simulink model "ATOM_planning_sim_variable_rear_ratio"  (R2026a)
settings: Solver=ode4  FixedStep=0.01
model workspace (MAT data in the model file):
  vehicle : object (value not decoded)
symbols that are objects in the model workspace (value not decoded): vehicle
undefined symbols (not defined in the file or in its folder): planning_validator, stanley, velocity_smoother
(part 2 of 4)

== matlab function ATOM_planning_sim_variable_rear_ratio/velocity_smoother_node/ApplySteeringRateLimit - velocity_smoother_node/Step2: Calculate steer rate for each trajectory point/ComputeSteeringRate4WS ==
  data: trajectory input Bus: TrajectoryDataBus; curvature input; veh input; steer_rate_velocity_ratio_arr output; points_interval input; output output Bus: TrajectoryDataBus
function [steer_rate_velocity_ratio_arr, output] = ComputeSteeringRateAngle4WS(trajectory, ...
    curvature, veh, ...
    points_interval)


% ComputeSteeringRateAngle4WS
%
% Computes steering angle rate ratio for 4WS.
%
% Equivalent to Autoware:
%
% steer_rate_velocity_ratio_arr
%
%
% The returned value represents:
%
%       steering_angle_difference / distance
%
%
% For 4WS:
%
% front and rear steering rates are computed.
%
% The maximum steering variation is used as constraint.

wheel_base = veh(3);
rear_steering_ratio = veh(29);

N = length(curvature);


front_angle = zeros(N,1);
rear_angle  = zeros(N,1);


%% Compute steering angles

for i = 1:N

    front_angle(i)= ...                                         % Modified for 4WS
        CalculateFrontSteeringAngle4WS( ...
        curvature(i), ...
        wheel_base, ...
        rear_steering_ratio);

    rear_angle(i) = rear_steering_ratio * front_angle(i);       % Modified for 4WS


    % This is a collateral effect of (&) in C++ when (considering in original
    % Autoware):
    %
    % auto & steer_front = output.at(i + 1).front_wheel_angle_rad;
    % auto & steer_back = output.at(i).front_wheel_angle_rad;
    % 
    % // calculate the just 2 steering angle
    % steer_front = std::atan(base_param_.wheel_base * curvature_v.at(i + 1));
    % steer_back = std::atan(base_param_.wheel_base * curvature_v.at(i));
    % Indeed, updating steer_front we popolate also output.at(i + 1).front_wheel_angle_rad, 
    % and so the output topic is populated (but it's just a collateral effect, front_wheel_angle_rad 
    % and rear_wheel_angle_rad contents are not important for Control module.

    trajectory.front_wheel_angle_rad(i) = front_angle(i);
    trajectory.rear_wheel_angle_rad(i) = rear_angle(i);

end




%% Compute steering rate

steer_rate_velocity_ratio_arr = zeros(N,1);


for i = 1:N-1


    % auto & steer_front = output.at(i + 1).front_wheel_angle_rad;
    % auto & steer_back = output.at(i).front_wheel_angle_rad;
    % const auto steering_diff = std::fabs(steer_front - steer_back);
    front_diff = abs( ...
        front_angle(i+1)-front_angle(i));


    rear_diff = abs( ...
        rear_angle(i+1)-rear_angle(i));


    steering_diff = max( ...                                    % Modified for 4WS --> conservative solution
        front_diff,...
        rear_diff);

    % eps avoids division by zero:
    eps = 2.220446049250313e-16;

    steer_rate_velocity_ratio_arr(i)= ...
        steering_diff/(points_interval+eps);


end


steer_rate_velocity_ratio_arr(end)= ...
    steer_rate_velocity_ratio_arr(end-1);


% Output topic now presents front_wheel_angle_rad and rear_wheel_angle_rad
% populated
output = trajectory;


end

== matlab function ATOM_planning_sim_variable_rear_ratio/velocity_smoother_node/ApplySteeringRateLimit - velocity_smoother_node/Step3: Remove noise by mean filter/MeanFilterSteeringRateRato ==
  data: steer_rate_ratio input; steer_rate_velocity_ratio_arr output
function steer_rate_velocity_ratio_arr = MeanFilterSteeringRateRatio( ...
    steer_rate_ratio)

% MeanFilterSteeringRateRatio
%
% Applies the same moving-average filter used by Autoware on the steering
% rate ratio.
%
% Equivalent to Step 3 inside:
%
%   SmootherBase::applySteeringRateLimit()
%
% in:
%
%   autoware_velocity_smoother
%
%
% Original C++ implementation:
%
% for (size_t i = 1; i < steer_rate_velocity_ratio_arr.size() - 1; i++) {
%
%   steer_rate_velocity_ratio_arr.at(i) =
%     (steer_rate_velocity_ratio_arr.at(i-1) +
%      steer_rate_velocity_ratio_arr.at(i)   +
%      steer_rate_velocity_ratio_arr.at(i+1))
%      / 3.0;
%
% }
%
%
% Notes
% -----
%
% The filter is performed in-place, exactly as in Autoware.
%
% Consequently, when computing sample i, the previous sample
% (i-1) has already been filtered, while the next sample (i+1)
% is still the original one.
%
% This behaviour is intentionally preserved to remain identical
% to the C++ implementation.


N = length(steer_rate_ratio);

steer_rate_velocity_ratio_arr = zeros(N,1);

for i = 2:N-1

    steer_rate_velocity_ratio_arr(i) = ...
        ( ...
        steer_rate_ratio(i-1) + ...
        steer_rate_ratio(i)   + ...
        steer_rate_ratio(i+1) ...
        ) / 3.0;

end


end

== matlab function ATOM_planning_sim_variable_rear_ratio/velocity_smoother_node/ApplySteeringRateLimit - velocity_smoother_node/ComputePointsInterval ==
  data: input_points_interval input; vel_smoother input; use_resampling input; points_interval output
function points_interval = computePointsInterval(input_points_interval, ...
    vel_smoother, use_resampling)

% Compute the trajectory points interval used for preprocessing.
%
% If resampling is enabled, a constant spatial interval is imposed.
% Otherwise, the original trajectory point spacing is preserved.

sample_ds = vel_smoother(3,1);

if use_resampling

    points_interval = sample_ds;

else

    points_interval = input_points_interval;

end

end

== matlab function ATOM_planning_sim_variable_rear_ratio/velocity_smoother_node/ApplySteeringRateLimit - velocity_smoother_node/ComputeIdxDist ==
  data: points_interval input; idx_dist output; vel_smoother input
function idx_dist = ComputeIdxDist( ...
    points_interval, ...
    vel_smoother)

% ComputeIdxDist
%
% Computes the point offset used for trajectory curvature estimation.
%
% The curvature is evaluated using three trajectory points separated by a
% fixed physical distance. Since the trajectory is sampled with a constant
% spatial interval (points_interval), this function converts the desired
% curvature calculation distance into the corresponding point index offset.
%
% In other words, idx_dist represents the number of trajectory points
% corresponding to the specified curvature calculation distance.
%
% Equivalent to the Autoware implementation:
%
% idx_dist = max(int(curvature_calculation_distance / points_interval), 1);

curvature_calculation_distance = vel_smoother(1);

idx_dist = max( ...
    floor(curvature_calculation_distance / points_interval), ...
    1);

== matlab function ATOM_planning_sim_variable_rear_ratio/velocity_smoother_node/ApplySteeringRateLimit - velocity_smoother_node/PlotTrajectoryCurvature ==
  data: trajectory input; curvature input
function PlotTrajectoryCurvature(trajectory, curvature)

% PlotTrajectoryCurvature
%
% Visualizes the trajectory curvature computed by:
%
%   ComputeTrajectoryCurvature()
%
% Equivalent to inspecting:
%
%   std::vector<double> k_arr
%
% generated inside:
%
%   autoware_motion_utils::calcTrajectoryCurvatureFrom3Points()
%
%
% Inputs
% -------
%
% trajectory:
%   MATLAB representation of Autoware TrajectoryPoints:
%
%       trajectory.pose.position.x
%       trajectory.pose.position.y
%
%
% curvature:
%   Nx1 signed curvature vector [1/m].
%
%   Positive curvature  -> left turn
%   Negative curvature  -> right turn


persistent hCurvature
persistent hTraj


%% Extract trajectory position

x = trajectory.pose.position.x;
y = trajectory.pose.position.y;


%% Check dimensions

if length(curvature) ~= length(x)

    error("Curvature vector length does not match trajectory length.");

end


%% Curvature profile

if isempty(hCurvature) 

    figure(3)
    clf

    hold on
    grid on

    hCurvature = plot( ...
        curvature, ...
        'LineWidth',1.5);


    xlabel("Trajectory point index");
    ylabel("Curvature [1/m]");

    title("Curvature profile");


else

    set(hCurvature,...
        'YData',curvature);

end



%% XY trajectory colored by curvature

if isempty(hTraj) 

    figure(4)
    clf

    hold on
    grid on
    axis equal


    hTraj = scatter( ...
        x, ...
        y, ...
        25, ...
        curvature, ...
        'filled');


    xlabel("x [m]");
    ylabel("y [m]");

    title("Trajectory curvature map");


    cb = colorbar;
    ylabel(cb,'Curvature [1/m]');


else

    set(hTraj,...
        'XData',x,...
        'YData',y,...
        'CData',curvature);

end


drawnow limitrate


end

== matlab function ATOM_planning_sim_variable_rear_ratio/velocity_smoother_node/ApplySteeringRateLimit - velocity_smoother_node/ComputeSteerRateVelocityRatioLimits ==
  data: velocity_thresholds input; steer_rate_velocity_ratio_limits output; steering_angle_rate_limits input
function steer_rate_velocity_ratio_limits = ...
    ComputeSteerRateVelocityRatioLimits( ...
    velocity_thresholds, ...
    steering_angle_rate_limits)

% ComputeSteerRateVelocityRatioLimits
%
% MATLAB equivalent of:
%
%   SmootherBase::computeSteerRateVelocityRatioLimits()
%
% in Autoware.
%
% It computes the steering-rate / velocity ratio limits used later by
% ComputeVelocityLimitFromSteerRate().
%
%
% Equivalent C++:
%
% return computeRatioLimits<double>(
%     velocity_thresholds,
%     steering_angle_rate_limits,
%     compute_steer_rate_ratio);
%
%
% Inputs
% -------
%
% velocity_thresholds
%       Velocity breakpoints [m/s]
%
% steering_angle_rate_limits
%       Maximum steering rate [deg/s]
%
%
% Output
% ------
%
% steer_rate_velocity_ratio_limits
%
% Nx2 matrix equivalent to:
%
% std::vector<std::pair<double,double>>
%
% Each row contains:
%
%   [ratio_lower , ratio_upper]
%
% corresponding to one velocity interval.


epsilon = 1e-5;

N = length(velocity_thresholds);

steer_rate_velocity_ratio_limits = zeros(N+1,2);


%% Compute ratio limits

for i = 1:N

    rate_deg = steering_angle_rate_limits(i);

    vi = velocity_thresholds(i);

    if i == 1
        vi_prev = 0.0;
    else
        vi_prev = velocity_thresholds(i-1);
    end

    steer_rate_velocity_ratio_limits(i,1) = ...
        deg2rad(rate_deg)/(vi_prev + epsilon);

    steer_rate_velocity_ratio_limits(i,2) = ...
        deg2rad(rate_deg)/(vi + epsilon);

end


%% Last interval

v_max = velocity_thresholds(end);

steer_rate_velocity_ratio_limits(end,1) = ...
    deg2rad(steering_angle_rate_limits(end)) / ...
    (v_max + epsilon);

steer_rate_velocity_ratio_limits(end,2) = 0.0;

end

== matlab function ATOM_planning_sim_variable_rear_ratio/velocity_smoother_node/MATLAB Function ==
  data: trajectory_input input; trajectory_output input; curvature input
function PlotSteeringRateVelocityLimit( ...
    trajectory_input, ...
    trajectory_output, ...
    curvature)

% PlotSteeringRateVelocityLimit
%
% Visualizes the velocity modification produced by the steering-rate
% velocity constraint.
%
% Equivalent to inspecting the difference between:
%
%   input.longitudinal_velocity_mps
%
% and:
%
%   output.longitudinal_velocity_mps
%
% after:
%
%   SmootherBase::applySteeringRateLimit()
%
% in Autoware.
%
%
% The steering-rate filter does not modify the trajectory geometry.
% It only reduces longitudinal velocity where the steering rate
% constraint is violated.
%
%
% Inputs
% -------
%
% trajectory_input:
%       Trajectory before ApplySteeringRateVelocityLimit()
%
%       Required fields:
%           trajectory.longitudinal_velocity_mps
%
%
% trajectory_output:
%       Trajectory after ApplySteeringRateVelocityLimit()
%
%       Required fields:
%           trajectory.longitudinal_velocity_mps
%
%
% curvature:
%       trajectory curvature [1/m]
%
%       Used only for visualization of curved regions.
%
%
% Output
% -------
%
% None
%
% Generates diagnostic plots:
%
%   - velocity before/after steering-rate constraint
%   - velocity reduction
%   - curvature profile


%% Extract velocities

vel_in = trajectory_input.longitudinal_velocity_mps;
vel_out = trajectory_output.longitudinal_velocity_mps;


N = length(vel_in);


if length(vel_out) ~= N
    error("Input and output trajectories have different lengths.");
end


%% Velocity variation

velocity_delta = vel_out - vel_in;


%% Plot velocity profile

persistent hVelIn hVelOut hCurvature hVelDelta1 hVelDelta2


if isempty(hVelIn)

    figure(5)
    hold on
    grid on

    hVelIn = plot( ...
        vel_in,...
        'LineWidth',1.5,...
        'DisplayName',"Input velocity");
    
    hVelOut = plot( ...
        vel_out,...
        '--',...
        'LineWidth',1.5,...
        'DisplayName',"After steering-rate limit");


    xlabel("Trajectory point index");
    ylabel("Longitudinal velocity [m/s]");
    
    title("Steering-rate velocity limitation");
    
    legend("Location","best");

else
    
    set(hVelIn, ...
        'YData', vel_in);
    
    set(hVelOut, ...
        'YData', vel_out);
end

%% Plot velocity reduction


if isempty(hVelDelta1)

    figure(6)
    hold on
    grid on

    hVelDelta1 = plot( ...
        velocity_delta,...
        'LineWidth',1.5);
    
    
    yline(0);
    
    
    xlabel("Trajectory point index");
    ylabel("\Delta velocity [m/s]");
    
    
    title("Velocity modification due to steering-rate constraint");

else

    set(hVelDelta1, ...
        'YData', velocity_delta);


end

drawnow limitrate

end

== matlab function ATOM_planning_sim_variable_rear_ratio/Demanded trajectory generation: Sinusoid 50m wavelength/Trajectory Generator: sinusoid ==
  data: x output; y output; z output; qx output; qy output; qz output; qw output; longitudinal_velocity_mps output; lateral_velocity_mps output; acceleration_mps2 output; heading_rate_rps output; front_wheel_angle_rad output; rear_wheel_angle_rad output
function [x,y,z,qx,qy,qz,qw,...
    longitudinal_velocity_mps,...
    lateral_velocity_mps,...
    acceleration_mps2,...
    heading_rate_rps,...
    front_wheel_angle_rad,...
    rear_wheel_angle_rad] = trajectoryGenerator

N = 100;

L = 100;                % trajectory length [m]
A = 5;                  % sinusoid amplitude [m]

x = linspace(0,L,N)';
y = A*sin(2*pi*x/50);      % wavelength = 50 m

z = zeros(N,1);

qx = zeros(N,1);
qy = zeros(N,1);
qz = zeros(N,1);
qw = zeros(N,1);

longitudinal_velocity_mps = 15*ones(N,1);

lateral_velocity_mps = zeros(N,1);
acceleration_mps2    = zeros(N,1);
heading_rate_rps     = zeros(N,1);

front_wheel_angle_rad = zeros(N,1);
rear_wheel_angle_rad  = zeros(N,1);

%% Orientation

dy = gradient(y,x);

yaw = atan(dy);

qz = sin(yaw/2);
qw = cos(yaw/2);

end

== matlab function ATOM_planning_sim_variable_rear_ratio/Demanded trajectory generation: 90° left turn/Trajectory Generator: 90° left turn ==
  data: x output; y output; z output; qx output; qy output; qz output; qw output; longitudinal_velocity_mps output; lateral_velocity_mps output; acceleration_mps2 output; heading_rate_rps output; front_wheel_angle_rad output; rear_wheel_angle_rad output
function [x,y,z,qx,qy,qz,qw,...
          longitudinal_velocity_mps,...
          lateral_velocity_mps,...
          acceleration_mps2,...
          heading_rate_rps,...
          front_wheel_angle_rad,...
          rear_wheel_angle_rad] = trajectoryGenerator

N = 100;

%% Geometry

R = 8;              % curve radius [m]

N1 = 30;            % first straight
N2 = 40;            % circular arc
N3 = 30;            % second straight


%% Allocate outputs

x = zeros(N,1);
y = zeros(N,1);
z = zeros(N,1);

qx = zeros(N,1);
qy = zeros(N,1);
qz = zeros(N,1);
qw = zeros(N,1);

longitudinal_velocity_mps = 15*ones(N,1);

lateral_velocity_mps = zeros(N,1);
acceleration_mps2 = zeros(N,1);
heading_rate_rps = zeros(N,1);

front_wheel_angle_rad = zeros(N,1);
rear_wheel_angle_rad = zeros(N,1);


%% ------------------------------------------------------------------------
%% First straight
%% ------------------------------------------------------------------------

L1 = 15;

for i = 1:N1

    t = (i-1)/(N1-1);

    x(i) = t*L1;
    y(i) = 0;

    yaw = 0;

    qz(i) = sin(yaw/2);
    qw(i) = cos(yaw/2);

end


%% ------------------------------------------------------------------------
%% Circular arc (90 deg)
%% ------------------------------------------------------------------------

center_x = L1;
center_y = R;

theta = linspace(-pi/2,0,N2);

for k = 1:N2

    i = N1+k;

    x(i) = center_x + R*cos(theta(k));
    y(i) = center_y + R*sin(theta(k));

    yaw = theta(k)+pi/2;

    qz(i) = sin(yaw/2);
    qw(i) = cos(yaw/2);

end


%% ------------------------------------------------------------------------
%% Second straight
%% ------------------------------------------------------------------------

L2 = 15;

x0 = x(N1+N2);
y0 = y(N1+N2);

for k = 1:N3

    i = N1+N2+k;

    t = k/(N3);

    x(i) = x0;
    y(i) = y0 + t*L2;

    yaw = pi/2;

    qz(i) = sin(yaw/2);
    qw(i) = cos(yaw/2);

end

end

== matlab function ATOM_planning_sim_variable_rear_ratio/trajectory_checker plugin - planning_validator_node/check_valid_steering/calcMaxSteeringAngles/calcSteeringAngles/calcCurvature ==
  data: trajectory input Bus: TrajectoryDataBus; curvature_vector output
function curvature_vector = ComputeTrajectoryCurvaturePlanningValidator(trajectory)

% ComputeTrajectoryCurvaturePlanningValidator
%
% Computes the trajectory curvature exactly as performed by the
% Autoware Planning Validator.
%
% Unlike VelocitySmoother, this implementation does NOT use idx_dist.
%
% Instead, for each trajectory point it searches the first previous and
% next trajectory points located at least:
%
%       curvature_distance = 1.0 [m]
%
% away along the trajectory arc length.
%
% The three selected points are then used by calcCurvature().
%
% This implementation reproduces:
%
% trajectory_checker_utils::calcCurvature()
%
% used inside:
%
% planning_validator
%
%
% Inputs
% -------
%
% trajectory
%
% MATLAB representation of Trajectory.
%
%
% Output
% -------
%
% curvature
%
% Nx1 curvature vector [1/m].

num_points = length(trajectory.pose.position.x);

curvature = zeros(num_points,1);

%% Need at least three points

if num_points < 3
    return
end

%% Arc-length computation

arc_length = zeros(num_points,1);

for i = 2:num_points

    dx = trajectory.pose.position.x(i) - ...
         trajectory.pose.position.x(i-1);

    dy = trajectory.pose.position.y(i) - ...
         trajectory.pose.position.y(i-1);

    ds = hypot(dx,dy);

    arc_length(i) = arc_length(i-1) + ds;

end

%% Curvature computation

curvature_distance = 1.0;      % [m]

first_distant_index = 0;
last_distant_index  = num_points;

for i = 2:num_points-1

    %% Search previous point

    idx_prev = 1;

    for j = i-1:-1:2

        if (arc_length(i)-arc_length(j)) > curvature_distance

            if first_distant_index == 0
                first_distant_index = i;
            end

            idx_prev = j;
            break

        end

    end

    %% Search next point

    idx_next = num_points;

    for j = i+1:num_points-1

        if (arc_length(j)-arc_length(i)) > curvature_distance

            last_distant_index = i;

            idx_next = j;
            break

        end

    end

    %% Extract points

    p1 = [
        trajectory.pose.position.x(idx_prev), ...
        trajectory.pose.position.y(idx_prev), ...
        trajectory.pose.position.z(idx_prev)
        ];

    p2 = [
        trajectory.pose.position.x(i), ...
        trajectory.pose.position.y(i), ...
        trajectory.pose.position.z(i)
        ];

    p3 = [
        trajectory.pose.position.x(idx_next), ...
        trajectory.pose.position.y(idx_next), ...
        trajectory.pose.position.z(idx_next)
        ];

    % In Autoware this call is wrapped inside a try/catch.
    % Since MATLAB code generation does not support exceptions,
    % calcCurvature() is assumed to always return a valid value.
    curvature(i) = calc_curvature(p1,p2,p3);

end

%% Replicate boundary values

% Equivalent to:
%
% for (size_t i = first_distant_index; i > 0; --i)
%   curvature(i-1)=curvature(i);

if first_distant_index > 0

    for i = first_distant_index:-1:2
        curvature(i-1) = curvature(i);
    end

end

% Equivalent to:
%
% for (size_t i = last_distant_index;
%      i < curvature.size()-1;
%      ++i)
%   curvature(i+1)=curvature(i);

if last_distant_index < num_points

    for i = last_distant_index:num_points-1
        curvature(i+1) = curvature(i);
    end

end

curvature_vector = curvature;

end

== matlab function ATOM_planning_sim_variable_rear_ratio/trajectory_checker plugin - planning_validator_node/check_valid_steering/calcMaxSteeringAngles/calcSteeringAngles/steering_vector calculation ==
  data: curvature input; front_steering_vector output; rear_steering_vector output; veh input
function [front_steering_vector, rear_steering_vector] = calcSteeringVector(curvature, veh)

wheel_base = veh(3);
rear_steering_ratio = veh(29);

N = length(curvature);

front_steering_vector = zeros(N,1);
rear_steering_vector  = zeros(N,1);

for i = 1:N

    front_steering_vector(i) = ...
        CalculateFrontSteeringAngle4WS( ...
        curvature(i),...
        wheel_base,...
        rear_steering_ratio);

    rear_steering_vector(i) = rear_steering_ratio*front_steering_vector(i);
    
end
    
end

== matlab function ATOM_planning_sim_variable_rear_ratio/trajectory_checker plugin - planning_validator_node/check_valid_steering/calcMaxSteeringAngles/GetAbsMaxValAndIdx front ==
  data: values input; max_value output; max_index output
function [max_value, max_index] = GetAbsMaxValAndIdx(values)

% GetAbsMaxValAndIdx
%
% Returns the maximum absolute value contained in the input vector and
% its corresponding index.
%
% Equivalent to:
%
% trajectory_checker_utils::getAbsMaxValAndIdx()
%
% in Autoware.
%
% C++ implementation:
%
% std::pair<double, size_t> getAbsMaxValAndIdx(...)
%
% which internally uses:
%
%   std::max_element(...)
%
% with the comparison:
%
%   abs(a) < abs(b)
%
%
% Inputs
% -------
%
% values
%     Nx1 vector.
%
%
% Outputs
% --------
%
% max_value
%     Maximum absolute value contained in the vector.
%
% max_index
%     Index of the element whose absolute value is maximum.
%
% Note
% ----
%
% MATLAB indices are 1-based, whereas the equivalent C++ implementation
% returns a 0-based index.

[max_value, max_index] = max(abs(values));

end

== matlab function ATOM_planning_sim_variable_rear_ratio/trajectory_checker plugin - planning_validator_node/check_valid_steering/calcMaxSteeringAngles/GetAbsMaxValAndIdx rear ==
  data: values input; max_value output; max_index output
function [max_value, max_index] = GetAbsMaxValAndIdx(values)

% GetAbsMaxValAndIdx
%
% Returns the maximum absolute value contained in the input vector and
% its corresponding index.
%
% Equivalent to:
%
% trajectory_checker_utils::getAbsMaxValAndIdx()
%
% in Autoware.
%
% C++ implementation:
%
% std::pair<double, size_t> getAbsMaxValAndIdx(...)
%
% which internally uses:
%
%   std::max_element(...)
%
% with the comparison:
%
%   abs(a) < abs(b)
%
%
% Inputs
% -------
%
% values
%     Nx1 vector.
%
%
% Outputs
% --------
%
% max_value
%     Maximum absolute value contained in the vector.
%
% max_index
%     Index of the element whose absolute value is maximum.
%
% Note
% ----
%
% MATLAB indices are 1-based, whereas the equivalent C++ implementation
% returns a 0-based index.

[max_value, max_index] = max(abs(values));

end

== matlab function ATOM_planning_sim_variable_rear_ratio/trajectory_checker plugin - planning_validator_node/check_valid_steering/calcMaxSteeringAngles/DecideValIdx ==
  data: max_steering output; max_index output; max_front input; idx_front input; max_rear input; idx_rear input
function [max_steering, max_index] = DecideValIdx(max_front, idx_front, ...
                                                  max_rear, idx_rear) 


if max_front >= max_rear

    max_steering = max_front;
    max_index    = idx_front;

else

    max_steering = max_rear;
    max_index    = idx_rear;

end

end

== matlab function ATOM_planning_sim_variable_rear_ratio/trajectory_checker plugin - planning_validator_node/check_valid_steering/CheckValidSteering ==
  data: max_steering input; is_valid_steering output; steering_threshold input
function is_valid_steering  = ...
    CheckValidSteering4WS( ...
    max_steering, steering_threshold)


% CheckValidSteering4WS
%
% Equivalent to:
%
% TrajectoryChecker::check_valid_steering()
%
% Autoware planning_validator
%
%
% The steering angle is NOT taken from:
%
%   trajectory.front_wheel_angle_rad
%   trajectory.rear_wheel_angle_rad
%
% Instead, Autoware recomputes it from trajectory geometry:
%
%   trajectory
%        |
%        v
%   curvature_vector
%        |
%        v
%   steering angle
%
%
% Adapted for 4WS:
%
% curvature =
%
%       (tan(delta_f)-tan(delta_r))/L
%
%
% where:
%
%       delta_r = rear_steering_ratio * delta_f
%
%
% Inputs
% -------
%
% trajectory:
%
%   trajectory.pose.position.x
%   trajectory.pose.position.y
%
%
% wheel_base:
%
%   vehicle wheelbase [m]
%
%
% rear_steering_ratio:
%
%   rear/front steering ratio
%
%
% steering_threshold:
%
%   maximum allowed steering angle [rad]
%
%
%
% Outputs
% --------
%
% is_valid_steering:
%
%   true  -> steering OK
%   false -> steering violation
%
%
% max_steering:
%
%   maximum absolute steering angle [rad]
%
%
% max_index:
%
%   trajectory point where maximum steering occurs
%
%
%

%% ============================================================
% Equivalent to:
%
% if (max_steering > params_.steering.threshold)
%
% =============================================================


if max_steering > steering_threshold

    is_valid_steering = false;

else

    is_valid_steering = true;

end


end

== matlab function ATOM_planning_sim_variable_rear_ratio/Vehicle Model/localization//kinematic_state function ==
  data: state input Bus: VehicleInternalStateBus; kinematic output Bus: KinematicStateBus; veh input
function kinematic = IntStateToKinematicState(state, veh)


%% Vehicle parameters

L = veh(3);


%% Current state

x = state.x;
y = state.y;
yaw = state.yaw;



% NOTE:
% vx is the longitudinal velocity expressed in the vehicle body frame
% (base_link located at the center of the rear axle).
% The vehicle speed magnitude is reconstructed as
%
%   v = vx / cos(delta_r)
%
% under the pure-rolling assumption (alpha_f = alpha_r = 0).

vx = state.vx;

steer_front = state.steer_front;
steer_rear  = state.steer_rear;


%% Pose

kinematic.pose.position.x = x;
kinematic.pose.position.y = y;
kinematic.pose.position.z = 0;


[qx,qy,qz,qw] = yawToQuaternion(yaw);

% quaternion from yaw only

kinematic.pose.orientation.x = qx;
kinematic.pose.orientation.y = qy;
kinematic.pose.orientation.z = qz;
kinematic.pose.orientation.w = qw;



%% Twist

% Body frame velocity

kinematic.twist.linear.x = vx;

kinematic.twist.linear.y = ...              % Modified for 4WS considering beta = steer_rear
    vx*tan(steer_rear);

kinematic.twist.linear.z = 0;



% Angular velocity

kinematic.twist.angular.x = 0;
kinematic.twist.angular.y = 0;

kinematic.twist.angular.z = ...
    vx/L * ...
    (tan(steer_front)-tan(steer_rear));


end

== matlab function ATOM_planning_sim_variable_rear_ratio/trajectory_checker plugin - planning_validator_node/check_valid_steering_rate/CheckValidSteeringRate ==
  data: max_steering_rate input; is_valid_steering_rate output; steering_rate_threshold input
function is_valid_steering_rate  = ...
    CheckValidSteering4WS( ...
    max_steering_rate, steering_rate_threshold)


% CheckValidSteering4WS
%
% Equivalent to:
%
% TrajectoryChecker::check_valid_steering()
%
% Autoware planning_validator
%
%
% The steering angle is NOT taken from:
%
%   trajectory.front_wheel_angle_rad
%   trajectory.rear_wheel_angle_rad
%
% Instead, Autoware recomputes it from trajectory geometry:
%
%   trajectory
%        |
%        v
%   curvature_vector
%        |
%        v
%   steering angle
%
%
% Adapted for 4WS:
%
% curvature =
%
%       (tan(delta_f)-tan(delta_r))/L
%
%
% where:
%
%       delta_r = rear_steering_ratio * delta_f
%
%
% Inputs
% -------
%
% trajectory:
%
%   trajectory.pose.position.x
%   trajectory.pose.position.y
%
%
% wheel_base:
%
%   vehicle wheelbase [m]
%
%
% rear_steering_ratio:
%
%   rear/front steering ratio
%
%
% steering_threshold:
%
%   maximum allowed steering angle [rad]
%
%
%
% Outputs
% --------
%
% is_valid_steering:
%
%   true  -> steering OK
%   false -> steering violation
%
%
% max_steering:
%
%   maximum absolute steering angle [rad]
%
%
% max_index:
%
%   trajectory point where maximum steering occurs
%
%
%

%% ============================================================
% Equivalent to:
%
% if (max_steering > params_.steering.threshold)
%
% =============================================================


if max_steering_rate > steering_rate_threshold

    is_valid_steering_rate = false;

else

    is_valid_steering_rate = true;

end


end

== matlab function ATOM_planning_sim_variable_rear_ratio/trajectory_checker plugin - planning_validator_node/check_valid_steering_rate/calcMaxSteeringRates/DecideValIdx ==
  data: max_steering_rate output; max_index output; max_front input; idx_front input; max_rear input; idx_rear input
function [max_steering_rate, max_index] = DecideValIdx(max_front, idx_front, ...
                                                  max_rear, idx_rear) 


if max_front >= max_rear

    max_steering_rate = max_front;
    max_index    = idx_front;

else

    max_steering_rate = max_rear;
    max_index    = idx_rear;

end

end

== matlab function ATOM_planning_sim_variable_rear_ratio/trajectory_checker plugin - planning_validator_node/check_valid_steering_rate/calcMaxSteeringRates/MATLAB Function ==
  data: trajectory input; max_steering_rate output; steering_vector input; max_index output
function [max_steering_rate, max_index] = ...
    CalcMaxSteeringRate(trajectory, steering_vector)


% CalcMaxSteeringRate
%
% Equivalent to:
%
% trajectory_checker_utils::calcMaxSteeringRates()
%
% in Autoware planning_validator.
%
%
% For 2WS:
%   steering_vector = front steering angle
%
% For 4WS:
%   call this function twice:
%
%   front_rate = CalcMaxSteeringRate(trajectory, front_vector)
%   rear_rate  = CalcMaxSteeringRate(trajectory, rear_vector)
%
% and take:
%
%   max(front_rate,rear_rate)
%
%
% Steering rate:
%
%       d(delta)/dt
%
% where:
%
%       dt = delta_s / velocity
%
%
% Units:
%
% steering_vector : [rad]
% trajectory velocity : [m/s]
% output : [rad/s]


N = length(steering_vector);


if N < 2

    max_steering_rate = 0;
    max_index = 1;

    return

end


max_steering_rate = 0;
max_index = 1;



for i = 1:N-1


    %% Distance between trajectory points

    dx = trajectory.pose.position.x(i+1) - ...
         trajectory.pose.position.x(i);

    dy = trajectory.pose.position.y(i+1) - ...
         trajectory.pose.position.y(i);


    delta_s = sqrt(dx^2 + dy^2);



    %% Mean velocity

    v = 0.5 * ( ...
        trajectory.longitudinal_velocity_mps(i+1) + ...
        trajectory.longitudinal_velocity_mps(i));



    %% Equivalent of:
    %
    % delta_s / max(v,1e-5)
    %
    % in C++

    dt = delta_s / max(v,1e-5);



    %% Steering rate

    steer_rate = ...
        (steering_vector(i+1)-steering_vector(i)) / dt;



    %% Equivalent of takeBigger()

    if abs(steer_rate) > max_steering_rate

        max_steering_rate = abs(steer_rate);

        max_index = i;

    end

end


end

== matlab function ATOM_planning_sim_variable_rear_ratio/trajectory_checker plugin - planning_validator_node/check_valid_steering_rate/calcMaxSteeringRates/MATLAB Function1 ==
  data: trajectory input; max_steering_rate output; steering_vector input; max_index output
function [max_steering_rate, max_index] = ...
    CalcMaxSteeringRate(trajectory, steering_vector)


% CalcMaxSteeringRate
%
% Equivalent to:
%
% trajectory_checker_utils::calcMaxSteeringRates()
%
% in Autoware planning_validator.
%
%
% For 2WS:
%   steering_vector = front steering angle
%
% For 4WS:
%   call this function twice:
%
%   front_rate = CalcMaxSteeringRate(trajectory, front_vector)
%   rear_rate  = CalcMaxSteeringRate(trajectory, rear_vector)
%
% and take:
%
%   max(front_rate,rear_rate)
%
%
% Steering rate:
%
%       d(delta)/dt
%
% where:
%
%       dt = delta_s / velocity
%
%
% Units:
%
% steering_vector : [rad]
% trajectory velocity : [m/s]
% output : [rad/s]


N = length(steering_vector);


if N < 2

    max_steering_rate = 0;
    max_index = 1;

    return

end


max_steering_rate = 0;
max_index = 1;



for i = 1:N-1


    %% Distance between trajectory points

    dx = trajectory.pose.position.x(i+1) - ...
         trajectory.pose.position.x(i);

    dy = trajectory.pose.position.y(i+1) - ...
         trajectory.pose.position.y(i);


    delta_s = sqrt(dx^2 + dy^2);



    %% Mean velocity

    v = 0.5 * ( ...
        trajectory.longitudinal_velocity_mps(i+1) + ...
        trajectory.longitudinal_velocity_mps(i));



    %% Equivalent of:
    %
    % delta_s / max(v,1e-5)
    %
    % in C++

    dt = delta_s / max(v,1e-5);



    %% Steering rate

    steer_rate = ...
        (steering_vector(i+1)-steering_vector(i)) / dt;



    %% Equivalent of takeBigger()

    if abs(steer_rate) > max_steering_rate

        max_steering_rate = abs(steer_rate);

        max_index = i;

    end

end


end

== matlab function ATOM_planning_sim_variable_rear_ratio/trajectory_checker plugin - planning_validator_node/check_valid_steering_rate/calcMaxSteeringRates/calcSteeringAngles/calcCurvature ==
  data: trajectory input Bus: TrajectoryDataBus; curvature_vector output
function curvature_vector = ComputeTrajectoryCurvaturePlanningValidator(trajectory)

% ComputeTrajectoryCurvaturePlanningValidator
%
% Computes the trajectory curvature exactly as performed by the
% Autoware Planning Validator.
%
% Unlike VelocitySmoother, this implementation does NOT use idx_dist.
%
% Instead, for each trajectory point it searches the first previous and
% next trajectory points located at least:
%
%       curvature_distance = 1.0 [m]
%
% away along the trajectory arc length.
%
% The three selected points are then used by calcCurvature().
%
% This implementation reproduces:
%
% trajectory_checker_utils::calcCurvature()
%
% used inside:
%
% planning_validator
%
%
% Inputs
% -------
%
% trajectory
%
% MATLAB representation of Trajectory.
%
%
% Output
% -------
%
% curvature
%
% Nx1 curvature vector [1/m].

num_points = length(trajectory.pose.position.x);

curvature = zeros(num_points,1);

%% Need at least three points

if num_points < 3
    return
end

%% Arc-length computation

arc_length = zeros(num_points,1);

for i = 2:num_points

    dx = trajectory.pose.position.x(i) - ...
         trajectory.pose.position.x(i-1);

    dy = trajectory.pose.position.y(i) - ...
         trajectory.pose.position.y(i-1);

    ds = hypot(dx,dy);

    arc_length(i) = arc_length(i-1) + ds;

end

%% Curvature computation

curvature_distance = 1.0;      % [m]

first_distant_index = 0;
last_distant_index  = num_points;

for i = 2:num_points-1

    %% Search previous point

    idx_prev = 1;

    for j = i-1:-1:2

        if (arc_length(i)-arc_length(j)) > curvature_distance

            if first_distant_index == 0
                first_distant_index = i;
            end

            idx_prev = j;
            break

        end

    end

    %% Search next point

    idx_next = num_points;

    for j = i+1:num_points-1

        if (arc_length(j)-arc_length(i)) > curvature_distance

            last_distant_index = i;

            idx_next = j;
            break

        end

    end

    %% Extract points

    p1 = [
        trajectory.pose.position.x(idx_prev), ...
        trajectory.pose.position.y(idx_prev), ...
        trajectory.pose.position.z(idx_prev)
        ];

    p2 = [
        trajectory.pose.position.x(i), ...
        trajectory.pose.position.y(i), ...
        trajectory.pose.position.z(i)
        ];

    p3 = [
        trajectory.pose.position.x(idx_next), ...
        trajectory.pose.position.y(idx_next), ...
        trajectory.pose.position.z(idx_next)
        ];

    % In Autoware this call is wrapped inside a try/catch.
    % Since MATLAB code generation does not support exceptions,
    % calcCurvature() is assumed to always return a valid value.
    curvature(i) = calc_curvature(p1,p2,p3);

end

%% Replicate boundary values

% Equivalent to:
%
% for (size_t i = first_distant_index; i > 0; --i)
%   curvature(i-1)=curvature(i);

if first_distant_index > 0

    for i = first_distant_index:-1:2
        curvature(i-1) = curvature(i);
    end

end

% Equivalent to:
%
% for (size_t i = last_distant_index;
%      i < curvature.size()-1;
%      ++i)
%   curvature(i+1)=curvature(i);

if last_distant_index < num_points

    for i = last_distant_index:num_points-1
        curvature(i+1) = curvature(i);
    end

end

curvature_vector = curvature;

end

== matlab function ATOM_planning_sim_variable_rear_ratio/trajectory_checker plugin - planning_validator_node/check_valid_steering_rate/calcMaxSteeringRates/calcSteeringAngles/steering_vector calculation ==
  data: curvature input; front_steering_vector output; rear_steering_vector output; veh input
function [front_steering_vector, rear_steering_vector] = calcSteeringVector(curvature, veh)

wheel_base = veh(3);
rear_steering_ratio = veh(29);

N = length(curvature);

front_steering_vector = zeros(N,1);
rear_steering_vector  = zeros(N,1);

for i = 1:N

    front_steering_vector(i) = ...
        CalculateFrontSteeringAngle4WS( ...
        curvature(i),...
        wheel_base,...
        rear_steering_ratio);

    rear_steering_vector(i) = rear_steering_ratio*front_steering_vector(i);
    
end
    
end

== matlab function ATOM_planning_sim_variable_rear_ratio/trajectory_checker plugin - planning_validator_node/HandleInvalidTrajectory - handling_type == default (case 0) ==
  data: trajectory_in input Bus: TrajectoryDataBus; trajectory_out output Bus: TrajectoryDataBus; is_valid_steering input; is_valid_steering_rate input
function trajectory_out  = ...
    HandleInvalidTrajectory( ...
    trajectory_in, ...
    is_valid_steering, ...
    is_valid_steering_rate)


% HandleInvalidTrajectory
%
% Equivalent to:
%
% PlanningValidatorNode::publishTrajectory()
%
% when:
%
% InvalidTrajectoryHandlingType::PUBLISH_AS_IT_IS
%
%
% If validation fails:
%
%   - trajectory is published unchanged
%   - validation status reports failure
%   - caution message is generated
%
%
% This reproduces Autoware behaviour.


%% ============================================================
% Validation status
% =============================================================

validation_status = ...
    is_valid_steering && is_valid_steering_rate;



%% ============================================================
% Publish trajectory behaviour
% =============================================================

% Default behaviour:
%
% PUBLISH_AS_IT_IS
%
% Therefore:
%
% output trajectory = input trajectory


trajectory_out = trajectory_in;



%% ============================================================
% Warning message
% =============================================================


if validation_status == false

     warning("Caution! Invalid Trajectory published.")

end


end

== matlab function ATOM_planning_sim_variable_rear_ratio/Demanded trajectory generation: 90° left turn critical for 2WS --> R = 2.4 m/Trajectory Generator: 90° left turn critical for 2WS ==
  data: x output; y output; z output; qx output; qy output; qz output; qw output; longitudinal_velocity_mps output; lateral_velocity_mps output; acceleration_mps2 output; heading_rate_rps output; front_wheel_angle_rad output; rear_wheel_angle_rad output
function [x,y,z,qx,qy,qz,qw,...
          longitudinal_velocity_mps,...
          lateral_velocity_mps,...
          acceleration_mps2,...
          heading_rate_rps,...
          front_wheel_angle_rad,...
          rear_wheel_angle_rad] = trajectoryGenerator

N = 100;

%% Geometry

R = 2.5;              % curve radius [m]

N1 = 30;            % first straight
N2 = 40;            % circular arc
N3 = 30;            % second straight


%% Allocate outputs

x = zeros(N,1);
y = zeros(N,1);
z = zeros(N,1);

qx = zeros(N,1);
qy = zeros(N,1);
qz = zeros(N,1);
qw = zeros(N,1);

longitudinal_velocity_mps = 15*ones(N,1);

lateral_velocity_mps = zeros(N,1);
acceleration_mps2 = zeros(N,1);
heading_rate_rps = zeros(N,1);

front_wheel_angle_rad = zeros(N,1);
rear_wheel_angle_rad = zeros(N,1);


%% ------------------------------------------------------------------------
%% First straight
%% ------------------------------------------------------------------------

L1 = 2;

for i = 1:N1

    t = (i-1)/(N1-1);

    x(i) = t*L1;
    y(i) = 0;

    yaw = 0;

    qz(i) = sin(yaw/2);
    qw(i) = cos(yaw/2);

end


%% ------------------------------------------------------------------------
%% Circular arc (90 deg)
%% ------------------------------------------------------------------------

center_x = L1;
center_y = R;

theta = linspace(-pi/2,0,N2);

for k = 1:N2

    i = N1+k;

    x(i) = center_x + R*cos(theta(k));
    y(i) = center_y + R*sin(theta(k));

    yaw = theta(k)+pi/2;

    qz(i) = sin(yaw/2);
    qw(i) = cos(yaw/2);

end


%% ------------------------------------------------------------------------
%% Second straight
%% ------------------------------------------------------------------------

L2 = 15;

x0 = x(N1+N2);
y0 = y(N1+N2);

for k = 1:N3

    i = N1+N2+k;

    t = k/(N3);

    x(i) = x0;
    y(i) = y0 + t*L2;

    yaw = pi/2;

    qz(i) = sin(yaw/2);
    qw(i) = cos(yaw/2);

end

end

== matlab function ATOM_planning_sim_variable_rear_ratio/Vehicle Model/Vehicle Dynamics/MATLAB Function ==
  data: state input Bus: VehicleInternalStateBus size=1; d_state output Bus: VehicleInternalStateBus size=1; command input Bus: ControlCMDBus size=1; veh input; rear_steering_command input
function d_state = vehicleDynamics(state, command, veh, rear_steering_command)

%%%%%%%%%%%%%%%%%%%%%%%%%%%%%%%%%%%%%%
%%%%%%%%%%%%%%%%%%%%%%%%%%%%%%%%%%%%%%
% Description:
% This vehicleDynamics model follows DELAY_STEER_ACC_GEARED
% model, it doesn't presents a model for gear management
% since its not something we're going to modify on Autoware for 4WS
% implementation.
%
% Inputs:
% - state: VehicleInternalStateBus. It contains the state of the vehicle
%          at time instant t. 
% - command: /control/command/control_cmd topic --> ControlCMDBus.
%          It contains the desired acc and steering commands coming from
%          the control region.
%
% - Parameters
% - vehicle: vehicle parameters struct defined in vehicleParameters.m.

% Outputs: 
% - d_state: It contains the derivative of the state of the vehicle at time
%          instant t+1.
%%%%%%%%%%%%%%%%%%%%%%%%%%%%%%%%%%%%%%
%%%%%%%%%%%%%%%%%%%%%%%%%%%%%%%%%%%%%%


% inside MATLAB Function: input is veh_in (1xN double)
v = veh; % 1xN numeric row

vehicle.param.wheel_radius    = v(1);
vehicle.param.wheel_width     = v(2);
vehicle.param.wheel_base      = v(3);
vehicle.param.wheel_tread     = v(4);
vehicle.param.front_overhang  = v(5);
vehicle.param.rear_overhang   = v(6);
vehicle.param.left_overhang   = v(7);
vehicle.param.right_overhang  = v(8);
vehicle.param.vehicle_height  = v(9);
vehicle.param.max_steer_angle = v(10);

% decode integer-coded enums (example)
vehicle.sim.vehicle_model_type = int32(v(11));    % or map to strings if needed
vehicle.sim.initialize_source  = int32(v(12));

vehicle.sim.timer_sampling_time_ms = v(13);
vehicle.sim.add_measurement_noise = logical(v(14));
vehicle.sim.vel_lim        = v(15);
vehicle.sim.vel_rate_lim   = v(16);
vehicle.sim.steer_lim      = v(17);
vehicle.sim.steer_rate_lim = v(18);
vehicle.sim.acc_time_delay = v(19);
vehicle.sim.acc_time_constant = v(20);
vehicle.sim.steer_time_delay   = v(21);
vehicle.sim.steer_time_constant= v(22);
vehicle.sim.x_stddev = v(23);
vehicle.sim.y_stddev = v(24);
vehicle.sim.steer_dead_band = v(25);
vehicle.sim.steer_bias = v(26);
vehicle.sim.debug_acc_scaling_factor = v(27);
vehicle.sim.debug_steer_scaling_factor = v(28);

% Parameter for 4WS
vehicle.param.rear_steering_ratio = veh(29);
rear_steering_ratio = vehicle.param.rear_steering_ratio;

%% ==========================
% Saturation function
% ===========================

sat = @(val, upper, lower) min(max(val,lower),upper);



%% ==========================
% Current state
% ===========================

vx = sat( ...
    state.vx,...
    vehicle.sim.vel_lim,...
   -vehicle.sim.vel_lim);


acc = sat( ...
    state.acc,...
    vehicle.sim.vel_rate_lim,...
   -vehicle.sim.vel_rate_lim);


yaw = state.yaw;

steer_front = state.steer_front;
steer_rear = state.steer_rear;          % Modified for 4WS  


%% ==========================
% Input commands
% ===========================

acc_des = sat( ...
    command.longitudinal.acceleration,...
    vehicle.sim.vel_rate_lim,...
   -vehicle.sim.vel_rate_lim);


acc_des = acc_des * ...
    vehicle.sim.debug_acc_scaling_factor;



steer_front_des = sat( ...
    command.lateral.steering_tire_angle,...
    vehicle.sim.steer_lim,...
   -vehicle.sim.steer_lim);


steer_front_des = steer_front_des * ...
    vehicle.sim.debug_steer_scaling_factor;

steer_rear_des = sat( ...                                            % Modified for 4WS
    rear_steering_command,...
    vehicle.sim.steer_lim,...
    -vehicle.sim.steer_lim);


steer_rear_des = steer_rear_des * ...                                % Modified for 4WS
    vehicle.sim.debug_steer_scaling_factor;



%% ==========================
% Steering dynamics
% ===========================

% getSteer() in simple_planning_simulator corresponds to state.steer
% From the phisical vehicle front_steer and rear_steer are measured.

steer_diff_front = steer_front - steer_front_des;

steer_diff_rear = steer_rear  - steer_rear_des;             % Modified for 4WS


% dead band

if steer_diff_front > vehicle.sim.steer_dead_band

    steer_diff_with_dead_band_front = ...
        steer_diff_front - vehicle.sim.steer_dead_band;


elseif steer_diff_front < -vehicle.sim.steer_dead_band

    steer_diff_with_dead_band_front = ...
        steer_diff_front + vehicle.sim.steer_dead_band;


else

    steer_diff_with_dead_band_front = 0;

end



if steer_diff_rear > vehicle.sim.steer_dead_band            % Modified for 4WS

    steer_diff_with_dead_band_rear = ...
        steer_diff_rear - vehicle.sim.steer_dead_band;


elseif steer_diff_rear < -vehicle.sim.steer_dead_band

    steer_diff_with_dead_band_rear = ...
        steer_diff_rear + vehicle.sim.steer_dead_band;


else

    steer_diff_with_dead_band_rear = 0;

end



steer_rate_front = sat( ...
    -steer_diff_with_dead_band_front / vehicle.sim.steer_time_constant,...
     vehicle.sim.steer_rate_lim,...
    -vehicle.sim.steer_rate_lim);

steer_rate_rear = sat( ...                                                  % Modified for 4WS
    -steer_diff_with_dead_band_rear / vehicle.sim.steer_time_constant,...
    vehicle.sim.steer_rate_lim,...
    -vehicle.sim.steer_rate_lim);



%% ==========================
% State derivative
% ===========================

%--------------------------------------------------------------
% 4WS kinematic bicycle model
%
% Assumptions:
%   - Pure rolling
%   - alpha_f = alpha_r = 0
%   - No tire dynamics
%   - No lateral slip dynamics
%
% beta is the geometric vehicle sideslip angle. Since Autoware defines
% reference frame of the vehicle equal to centre of the rear axle, then
% beta = steer_rear
%--------------------------------------------------------------

L = vehicle.param.wheel_base;


beta = steer_rear;                              % Modified for 4WS


vel = vx/cos(beta);                             % Modified for 4WS


yaw_rate = ...                                  % Modified for 4WS
    vx/L * ...
    (tan(steer_front)-tan(steer_rear));


d_state.x = vel*cos(yaw + beta);                % Modified for 4WS

d_state.y = vel*sin(yaw + beta);                % Modified for 4WS


d_state.yaw = yaw_rate;                         % Modified for 4WS


d_state.vx = acc;


d_state.steer_front = steer_rate_front;

d_state.steer_rear = steer_rate_rear;           % Modified for 4WS

d_state.acc = ...
    -(acc-acc_des)/vehicle.sim.acc_time_constant;

end

== matlab function ATOM_planning_sim_variable_rear_ratio/Lateral run()/RearToFrontOdometry ==
  data: rear_pose input Bus: KinematicStateBus; front_pose output Bus: KinematicStateBus; wheel_base input
function front_pose = RearToFrontOdometry( ...
    rear_pose,...
    wheel_base)


front_pose = rear_pose;


qx = rear_pose.pose.orientation.x;
qy = rear_pose.pose.orientation.y;
qz = rear_pose.pose.orientation.z;
qw = rear_pose.pose.orientation.w;


yaw = QuaternionToYaw(qx,qy,qz,qw);



front_pose.pose.position.x = ...
    rear_pose.pose.position.x + ...
    wheel_base*cos(yaw);


front_pose.pose.position.y = ...
    rear_pose.pose.position.y + ...
    wheel_base*sin(yaw);


front_pose.pose.position.z = ...
    rear_pose.pose.position.z;



% orientation unchanged

front_pose.pose.orientation = ...
    rear_pose.pose.orientation;


% Linear velocity referred to front axle

front_pose.twist.linear.x = rear_pose.twist.linear.x ...
    - rear_pose.twist.angular.z ...
    * wheel_base*sin(yaw);


front_pose.twist.linear.y = rear_pose.twist.linear.y ...
    + rear_pose.twist.angular.z ...
    * wheel_base*cos(yaw);


front_pose.twist.linear.z = rear_pose.twist.linear.z;


end
